simulink model "OBSERVADOR"  (Simulink 9.1)
settings: Solver=ode4  StartTime=0.0  StopTime=50  FixedStep=0.01  RelTol=1e-3  EnableMultiTasking=on
values from neighbouring files (symbols this model uses):
  g = 9.81    [parametros.m]
  ka = .02    (= 0.02)    [parametros.m]
  l = .23    (= 0.23)    [parametros.m]
  L1 = 2*zo*wno-ka/(m*l)    (= 35.8260869565)    [parametros.m]
  L2 = wno^2-L1*ka/(m*l)-g/l    (= 275.117202268)    [parametros.m]
  m = .5    (= 0.5)    [parametros.m]
libraries: fuzblock x1
settings Model: Creator=ULTIMATE HP  LastModifiedBy=Benjamin Nicolas
settings DataIOCC: LimitDataPoints=on  SignalLoggingSaveFormat=ModelDataLogs
settings OptimizationCC: ExpressionDepthLimit=2147483647
settings DebuggingCC: FcnCallInpInsideContextMsg=warning  StateNameClashWarn=warning
settings GRTTargetCC: GeneratePreprocessorConditionals=Disable all

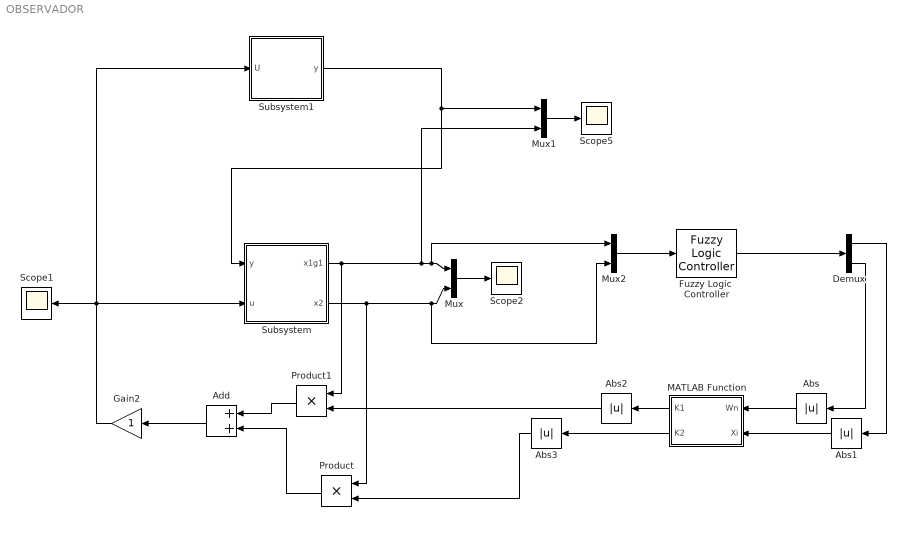
== system OBSERVADOR ==
  Abs{,1..3} (4 alike) : Abs
  Add : Sum
  Demux : Demux  Outputs=2
  Fuzzy Logic  Controller : fuzblock/Fuzzy Logic  Controller  FIS=OBSE  OutputSampleNumber=101  DataType=double  FuzzifiedInputs=off  RuleFiringStrengths=off  RuleOutputs=off  AggregatedOutputs=off  SimulateUsing=Interpreted execution
  Gain2 : Gain
  MATLAB Function : MATLAB Function  TreatAsAtomicUnit=on
  Mux : Mux  Inputs=2
  Mux1 : Mux  Inputs=2
  Mux2 : Mux  Inputs=2
  Product : Product  RndMeth=Zero
  Product1 : Product  RndMeth=Zero
  Scope1 : Scope
  Scope2 : Scope
  Scope5 : Scope
  Subsystem : Subsystem
  Subsystem1 : Subsystem
  wires:
  Subsystem1/1("y ") -> Mux1/1, Subsystem/1("y ")
  Add/1 -> Gain2/1
  Gain2/1 -> Subsystem1/1(U), Scope1/1, Subsystem/2("u ")
  Mux/1 -> Scope2/1
  Subsystem/1(x1g1) -> Mux1/2, Mux/1, Mux2/1, Product1/1
  Subsystem/2("x2 ") -> Mux/2, Mux2/2, Product/1
  Mux1/1 -> Scope5/1
  Mux2/1 -> Fuzzy Logic  Controller/1
  Product1/1 -> Add/1
  Product/1 -> Add/2
  MATLAB Function/1(K1) -> Abs2/1
  MATLAB Function/2(K2) -> Abs3/1
  Fuzzy Logic  Controller/1 -> Demux/1
  Demux/1 -> Abs1/1
  Demux/2 -> Abs/1
  Abs/1 -> MATLAB Function/1(Wn)
  Abs1/1 -> MATLAB Function/2(Xi)
  Abs2/1 -> Product1/2
  Abs3/1 -> Product/2

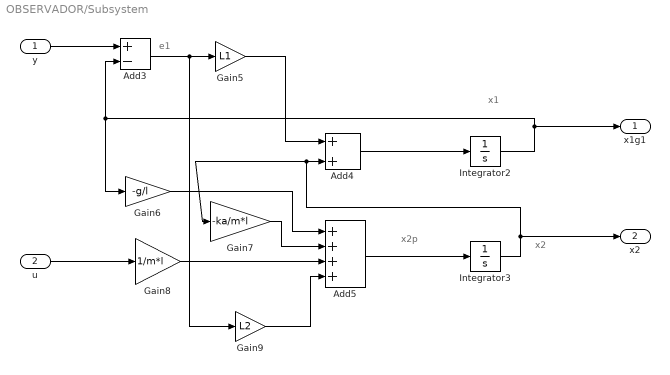
== system OBSERVADOR/Subsystem ==
  note: x2p
  note: x2
  note: x1
  note: e1
  "y " : Inport
  "u " : Inport  Port=2
  Add3 : Sum  Inputs=+-
  Add4 : Sum
  Add5 : Sum  Inputs=++++
  Gain5 : Gain  Gain=L1
  Gain6 : Gain  Gain=-g/l
  Gain7 : Gain  Gain=-ka/m*l
  Gain8 : Gain  Gain=1/m*l
  Gain9 : Gain  Gain=L2
  Integrator2 : Integrator
  Integrator3 : Integrator
  x1g1 : Outport
  "x2 " : Outport  Port=2
  wires:
  "u "/1 -> Gain8/1
  Gain9/1 -> Add5/4
  Integrator2/1 -> x1g1/1, Add3/2, Gain6/1
  Gain5/1 -> Add4/1
  Gain8/1 -> Add5/3
  Gain7/1 -> Add5/2
  Add4/1 -> Integrator2/1
  Add5/1 -> Integrator3/1
  Integrator3/1 -> "x2 "/1, Add4/2, Gain7/1
  Add3/1 -> Gain9/1, Gain5/1
  Gain6/1 -> Add5/1
  "y "/1 -> Add3/1

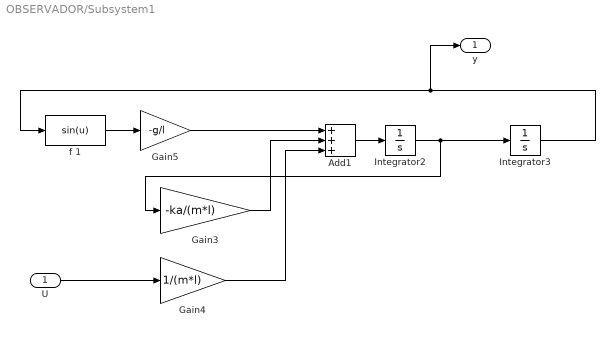
== system OBSERVADOR/Subsystem1 ==
  U : Inport
  Add1 : Sum  Inputs=+++
  Gain3 : Gain  Gain=-ka/(m*l)
  Gain4 : Gain  Gain=1/(m*l)
  Gain5 : Gain  Gain=-g/l
  Integrator2 : Integrator
  Integrator3 : Integrator  InitialCondition=pi/2
  f 1 : Fcn  Expr=sin(u)
  "y " : Outport
  wires:
  f 1/1 -> Gain5/1
  Integrator3/1 -> "y "/1, f 1/1
  U/1 -> Gain4/1
  Gain3/1 -> Add1/2
  Gain4/1 -> Add1/3
  Add1/1 -> Integrator2/1
  Integrator2/1 -> Gain3/1, Integrator3/1
  Gain5/1 -> Add1/1

== matlab function MATLAB Function ==
  data: Wn input double; K1 output double; Xi input double; K2 output double
function [K1, K2] = fcn(Wn, Xi)
m =.5;
l =.23;
ka =.02;
g = 9.81;
L1=2*Xi*Wn-ka/(m*l);
L2=Wn^2-L1*ka/(m*l)-g/l
K1=g/l-Wn^2;
K2=ka/(m*l)-2* Xi*Wn;
%y = u;
